simulink model "homework6_1"  (R2023a)
settings: Solver=VariableStepAuto  StartTime=0.0  StopTime=5  RelTol=1e-3
libraries: spsVoltageMeasurementLib x4, spsAsynchronousMachineSIUnitsLib x1, spsDCVoltageSourceLib x1, spsGroundLib x1, simulink x1, spsThreePhaseProgrammableVoltageSourceLib x1, spsUniversalBridgeLib x1, sps_lib x1
settings Model: Creator=zou20  LastModifiedBy=zou20

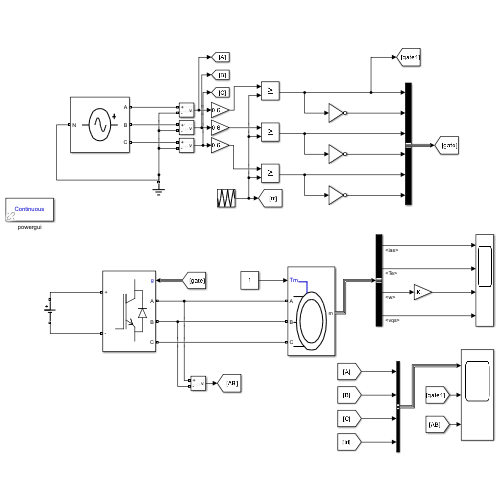
[thumbnail: Simulink's stored preview of the top-level diagram]
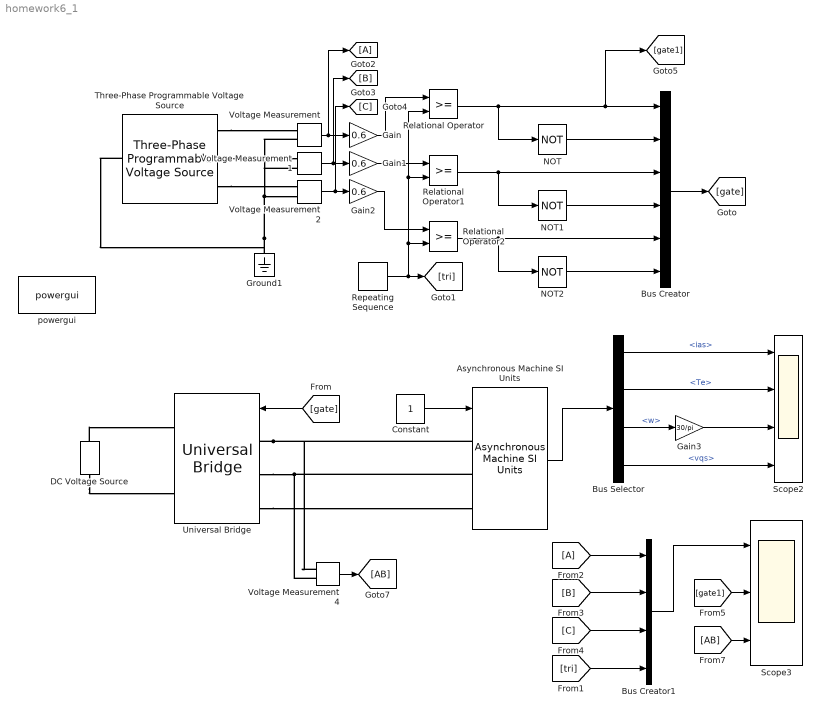
== system homework6_1 ==
  Asynchronous Machine SI Units : spsAsynchronousMachineSIUnitsLib/Asynchronous Machine SI Units  RotorType=Squirrel-cage  PresetModel=No  MechanicalLoad=Torque Tm  ShowDetailedParameters=on  ReferenceFrame=Rotor  Units=SI  MeasurementBus=on  NominalParameters=[1.845e+04 400 50]  VoltageRatio=1  Stator=[0.5968 0.0003495]  Rotor=[0.6258 0.005473]  Cage1=[0.4155 0.002066]  Cage2=[0.4168 0.0003495]  Lm=0.0354  Mechanical=[0.05 0.005879 2]  PolePairs=2  InitialConditions=[0 0 0 0 0 0 0 0]  SimulateSaturation=off  Saturation=[14.03593122, 27.81365428, 53.79336849, 72.68890987, 97.98006896, 148.6815601, 215.7428561, 302.9841135, 428.7778367 ; 230, 322, 414, 460, 506, 552, 598, 644, 690]  LoadFlowParameters=1492000  TsPowergui=0  TsBlock=-1  IterativeModel=Trapezoidal non iterative  IterativeDiscreteModel=Trapezoidal non iterative  Pmec=1.492e+006
  Bus Creator : BusCreator  Inputs=6
  Bus Creator1 : BusCreator  Inputs=4
  Bus Selector : BusSelector  OutputSignals=ias,Te,w,vqs
  Constant : Constant
  DC Voltage Source : spsDCVoltageSourceLib/DC Voltage Source  Amplitude=100  Measurements=None
  From2 : From
  Gain : Gain  Gain=0.6
  Gain1 : Gain  Gain=0.6
  Gain2 : Gain  Gain=0.6
  Gain3 : Gain  Gain=30/pi
  Goto2 : Goto
  Ground1 : spsGroundLib/Ground  LConnTagsString=a
  NOT : Logic  Operator=NOT  IconShape=distinctive  AllPortsSameDT=off  OutDataTypeStr=boolean
  NOT1 : Logic  Operator=NOT  IconShape=distinctive  AllPortsSameDT=off  OutDataTypeStr=boolean
  NOT2 : Logic  Operator=NOT  IconShape=distinctive  AllPortsSameDT=off  OutDataTypeStr=boolean
  Relational Operator : RelationalOperator  OutDataTypeStr=boolean  RndMeth=Simplest  InputSameDT=off
  Relational Operator1 : RelationalOperator  OutDataTypeStr=boolean  RndMeth=Simplest  InputSameDT=off
  Relational Operator2 : RelationalOperator  OutDataTypeStr=boolean  RndMeth=Simplest  InputSameDT=off
  Repeating Sequence : simulink/Sources/Repeating Sequence  rep_seq_t=[0/500 0.125/500 0.25/500 0.375/500 0.5/500]  rep_seq_y=[0 -1 0 1 0]
  Scope2 : Scope  NumInputPorts=4
  Scope3 : Scope  NumInputPorts=3
  Three-Phase Programmable Voltage Source : spsThreePhaseProgrammableVoltageSourceLib/Three-Phase Programmable Voltage Source  PositiveSequence=[1 0 50]  VariationEntity=None  VariationType=Table of time-amplitude pairs  VariationTypeAlt=Step  VariationStep=0.5  VariationRate=10  VariationMagnitude=0.3  VariationFrequency=2  VariationTiming=[1 2]  VariationPhaseA=off  Amplitudes=[1 0.8 1.2 1.0]  TimeValues=[0 0.1 0.15 0.2]  HarmonicGeneration=off  HarmonicA=[3 0.2 -25 0]  HarmonicB=[2 0.15 35 2]  Timing="[0.05  3]"  BusType=swing  Pref=0  Qref=0  Qmin=-inf  Qmax=inf
  Universal Bridge : spsUniversalBridgeLib/Universal Bridge  Arms=3  SnubberResistance=1e5  SnubberCapacitance=inf  Device=IGBT / Diodes  Ron=1e-3  Lon=0  ForwardVoltages="[  0  0  ]"  ForwardVoltage=0  GTOparameters=[ 10e-6 , 20e-6 ]  IGBTparameters=[ 1e-6 , 2e-6 ]  Measurements=None  Measurements_2=None  converterType=Rectifier
  Voltage Measurement{,1..2,4} (4 alike) : spsVoltageMeasurementLib/Voltage Measurement  PhasorSimulation=off  OutputType=Complex  PSBequivalent=0
  powergui : sps_lib/powergui  Priority=1  SimulationMode=Continuous  SampleTime=50e-6  frequency=60  Iterations=50  frequencyindice=50  Pbase=100e6  ErrMax=1e-4  UnitsV=kV  UnitsW=MW  buscounter=0  FunctionMessages=off  echomessages=off  EnableUseOfTLC=off  CurrentSourceSwitches=off  DisableSnubberDevices=off  DisableRonSwitches=off  DisableVfSwitches=off  DisplayEquations=off  AutomaticDiscreteSolvers=off  SolverType=Tustin/Backward Euler (TBE)  Interpol=off  ExternalGateDelay=off  methode=off  Ts=100  x0status=blocks  SPID=on  SwTol=0  HookPort=off  NonlinearTolerance=1e-4  nMaxIteration=100  ContinueOnMaxIteration=off  RestoreLinks=warning  ResistiveCurrentMeasurement=off  Frange=[0:2:500]  Ylog=off  Xlog=on  ShowGrid=off  save=off  variable=ZData  structure=0  ZoomFFT=off  StartTime=0.0  cycles=1  DisplayStyle=1  fundamental=60  FreqAxis=off  MaxFrequency=1000  frequencyindicesteady=1  RmsSteady=1  display=off
  wires:
  Voltage Measurement/1 -> Goto2/1, Gain/1
  Voltage Measurement1/1 -> [B], Gain1/1
  Voltage Measurement2/1 -> [C], Gain2/1
  Gain/1 -> Relational Operator/1
  Gain1/1 -> Relational Operator1/1
  Gain2/1 -> Relational Operator2/1
  Repeating Sequence/1 -> Relational Operator/2, Relational Operator1/2, Relational Operator2/2, [tri]
  Relational Operator/1 -> [gate1], Bus Creator/1, NOT/1
  Relational Operator1/1 -> Bus Creator/3, NOT1/1
  Relational Operator2/1 -> Bus Creator/5, NOT2/1
  NOT/1 -> Bus Creator/2
  NOT1/1 -> Bus Creator/4
  NOT2/1 -> Bus Creator/6
  Bus Creator/1 -> [gate]
  [tri] -> Bus Creator1/4
  [C] -> Bus Creator1/3
  [B] -> Bus Creator1/2
  From2/1 -> Bus Creator1/1
  Bus Selector/1 -> Scope2/1  "<ias>"
  Bus Selector/2 -> Scope2/2  "<Te>"
  Constant/1 -> Asynchronous Machine SI Units/1
  [gate] -> Universal Bridge/1
  Bus Selector/3 -> Gain3/1  "<w>"
  Asynchronous Machine SI Units/1 -> Bus Selector/1
  Bus Selector/4 -> Scope2/4  "<vqs>"
  Bus Creator1/1 -> Scope3/1
  [gate1] -> Scope3/2
  Voltage Measurement4/1 -> [AB]
  [AB] -> Scope3/3
  Gain3/1 -> Scope2/3
  connections:
  Three-Phase Programmable Voltage Source/RConn1 -- Voltage Measurement/LConn1
  Three-Phase Programmable Voltage Source/RConn2 -- Voltage Measurement1/LConn1
  Three-Phase Programmable Voltage Source/RConn3 -- Voltage Measurement2/LConn1
  Ground1/LConn1 -- Voltage Measurement/LConn2 -- Voltage Measurement1/LConn2 -- Voltage Measurement2/LConn2 -- Three-Phase Programmable Voltage Source/LConn1
  Universal Bridge/LConn3 -- Asynchronous Machine SI Units/LConn3
  Asynchronous Machine SI Units/LConn2 -- Universal Bridge/LConn2 -- Voltage Measurement4/LConn2
  DC Voltage Source/RConn1 -- Universal Bridge/RConn1
  Universal Bridge/LConn1 -- Asynchronous Machine SI Units/LConn1 -- Voltage Measurement4/LConn1
  DC Voltage Source/LConn1 -- Universal Bridge/RConn2
